simulink model "dspwavelet_frame"  (Simulink 8.3)
settings: Solver=FixedStepDiscrete  StartTime=0.0  StopTime=1024  RelTol=1e-3
model workspace: external: MAT-File dspwlets.mat (data not in the file)
undefined symbols (not defined in the file or in its folder): lod, ts
libraries: dspsigops x5, dspmlti4 x4, dspstat3 x2, simulink x2, dspmisc x1, dspsrcs4 x1
settings Model: Creator=The MathWorks Inc.  ExtModeTrigMode=oneshot  ExtModeArmWhenConnect=off
settings DataIOCC: LimitDataPoints=off  SaveOutput=off  SaveTime=off  SignalLoggingName=sigsOut
settings OptimizationCC: BlockReduction=off  BooleanDataType=off  ExpressionDepthLimit=2147483647  InitFltsAndDblsToZero=on  EfficientMapNaN2IntZero=off
settings DebuggingCC: SaveWithParameterizedLinksMsg=none  SignalResolutionControl=TryResolveAllWithWarning  SolverPrmCheckMsg=none  MultiTaskDSMMsg=warning  MultiTaskCondExecSysMsg=none  IntegerOverflowMsg=none  FcnCallInpInsideContextMsg=UseLocalSettings  StrictBusMsg=None
settings HardwareCC: TargetUnknown=on
settings RTWCC: IncludeERTFirstTime=on
settings GRTTargetCC: TargetFcnLib=ansi_tfl_tmw.mat

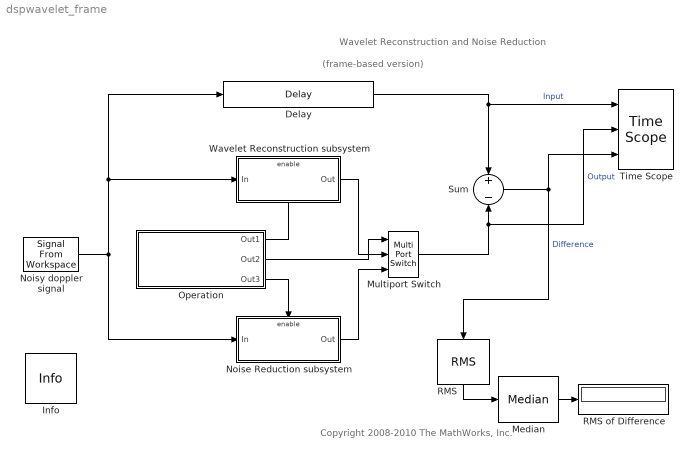
== system dspwavelet_frame ==
  note: Wavelet Reconstruction and Noise Reduction
  note: Copyright 2008-2010 The MathWorks, Inc.
  note: (frame-based version)
  Delay : dspsigops/Delay  InputProcessing=Columns as channels (frame based)  dly_unit=Samples  delay=7*(length(lod)-1)  ic_detail=on  dif_ic_for_ch=off  dif_ic_for_dly=off  ic=0  reset_popup=None
  Info : dspmisc/Info  SystemSampleTime=-1
  Median : dspstat3/Median  sortAlg=Quick sort  directionMode=Each column  dimension=1  treatSBRowAsCol=on  outputDataTypeStr=Inherit: Same as accumulator  outputLastDataTypeStr=Inherit: Same as accumulator  outputMin=[]  outputMax=[]  accumDataTypeStr=Inherit: Same as product output  accumLastDataTypeStr=Inherit: Same as product output  roundingMode=Floor  overflowMode=off
      settings: allowOverrides=off
  Multiport Switch : MultiPortSwitch  DataPortOrder=Zero-based contiguous  Inputs=2  zeroidx=on
  Noise Reduction subsystem : Subsystem  TreatAsAtomicUnit=on
  Noisy doppler signal : dspsrcs4/Signal From Workspace  X=noisdopp  Ts=ts  nsamps=64  OutputAfterFinalValue=Setting to zero  ignoreOrWarnInputAndFrameLengths=off
  Operation : Subsystem  mask(Wavelet Application){operation=Remove noise}
      mask help: Select a wavelet application
      mask init:
      | if operation == 1
      |     str = 'Perfect Reconstruction';
      | else
      |     str = 'Remove Noise';
      | end
      mask TypeOptions operation: Perfect reconstruction | Remove noise
      mask Display: disp(str)
  RMS : dspstat3/RMS  run=on  reset_popup=None  InputProcessing=Columns as channels (frame based)  directionMode=Entire input  dimension=1  treatSBRowAsCol=on
  RMS of Difference : Display
  Sum : Sum  Inputs=+-  SaturateOnIntegerOverflow=on  InputSameDT=on  OutDataTypeStr=Inherit: Same as first input
  Time Scope : TimeScope  NumInputPorts=3  DefaultConfigurationName=spbscopes.TimeScopeBlockCfg  ScopeSpecification=DataTag4
  Wavelet Reconstruction subsystem : Subsystem  TreatAsAtomicUnit=on
  wires:
  Delay/1 -> Sum/1, Time Scope/1  "Input"
  Sum/1 -> RMS/1, Time Scope/3  "Difference"
  Operation/1(Out1) -> Wavelet Reconstruction subsystem/Enable
  Noisy doppler signal/1 -> Noise Reduction subsystem/1(In), Delay/1, Wavelet Reconstruction subsystem/1(In)
  Operation/2(Out2) -> Multiport Switch/1
  Operation/3(Out3) -> Noise Reduction subsystem/Enable
  Noise Reduction subsystem/1(Out) -> Multiport Switch/3
  Multiport Switch/1 -> Time Scope/2, Sum/2  "Output"
  RMS/1 -> Median/1
  Wavelet Reconstruction subsystem/1(Out) -> Multiport Switch/2
  Median/1 -> RMS of Difference/1

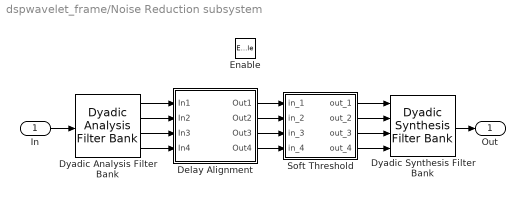
== system dspwavelet_frame/Noise Reduction subsystem ==
  In : Inport
  Enable : EnablePort
  Delay Alignment : Subsystem
  Dyadic Analysis Filter Bank : dspmlti4/Dyadic Analysis Filter Bank  Wname=User-defined  OrdRec_ordDec=[1 / 1]  Order=2  LPF=lod  HPF=hid  NumLevels=3  tree=Asymmetric  Output=Multiple ports
  Dyadic Synthesis Filter Bank : dspmlti4/Dyadic Synthesis Filter Bank  Wname=User-defined  OrdRec_ordDec=[1 / 1]  Order=2  LPF=lor  HPF=hir  NumLevels=3  tree=Asymmetric  Input=Multiple ports
  Soft Threshold : Subsystem  mask(Soft Threshold){st=[3 2 1 0]}
      mask prompts: st "Vector of thresholds for each level:"
      mask help: Apply a soft threshold (deadzone transfer function) to each signal in the decomposition. First threshold applies to top-most filter bank output.
      mask init:
      | x=([-1 1 NaN 0 0 NaN -1 -.5 .5 1]+1)/2*.7+.15;
      | y=([0 0 NaN -1 1 NaN -1 0 0 1]+1)/2*.7+.05;
      mask Help: Vector of thresholds for each decomposition level.
      mask Display:
      | text(.1,.9,'Dead Zone')
      | plot(x,y)
  Out : Outport
  wires:
  In/1 -> Dyadic Analysis Filter Bank/1
  Dyadic Synthesis Filter Bank/1 -> Out/1
  Dyadic Analysis Filter Bank/2 -> Delay Alignment/2(In2)
  Dyadic Analysis Filter Bank/1 -> Delay Alignment/1(In1)
  Delay Alignment/2(Out2) -> Soft Threshold/2(in_2)
  Delay Alignment/1(Out1) -> Soft Threshold/1(in_1)
  Soft Threshold/1(out_1) -> Dyadic Synthesis Filter Bank/1
  Soft Threshold/2(out_2) -> Dyadic Synthesis Filter Bank/2
  Dyadic Analysis Filter Bank/3 -> Delay Alignment/3(In3)
  Dyadic Analysis Filter Bank/4 -> Delay Alignment/4(In4)
  Delay Alignment/3(Out3) -> Soft Threshold/3(in_3)
  Delay Alignment/4(Out4) -> Soft Threshold/4(in_4)
  Soft Threshold/3(out_3) -> Dyadic Synthesis Filter Bank/3
  Soft Threshold/4(out_4) -> Dyadic Synthesis Filter Bank/4

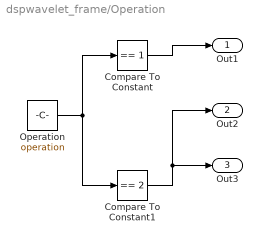
== system dspwavelet_frame/Operation ==
  Compare To Constant : simulink/Logic and Bit Operations/Compare To Constant  relop===  const=1  OutDataTypeStr=uint8  ZeroCross=off
  Compare To Constant1 : simulink/Logic and Bit Operations/Compare To Constant  relop===  const=2  OutDataTypeStr=uint8  ZeroCross=off
  Operation : Constant  Value=operation
  Out1 : Outport
  Out2 : Outport  Port=2
  Out3 : Outport  Port=3
  wires:
  Operation/1 -> Compare To Constant/1, Compare To Constant1/1
  Compare To Constant/1 -> Out1/1
  Compare To Constant1/1 -> Out3/1, Out2/1

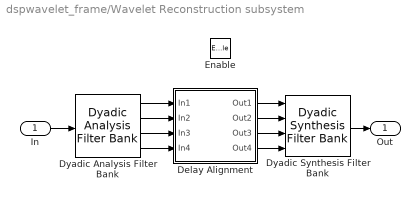
== system dspwavelet_frame/Wavelet Reconstruction subsystem ==
  In : Inport
  Enable : EnablePort
  Delay Alignment : Subsystem
  Dyadic Analysis Filter Bank : dspmlti4/Dyadic Analysis Filter Bank  Wname=User-defined  OrdRec_ordDec=[1 / 1]  Order=2  LPF=lod  HPF=hid  NumLevels=3  tree=Asymmetric  Output=Multiple ports
  Dyadic Synthesis Filter Bank : dspmlti4/Dyadic Synthesis Filter Bank  Wname=User-defined  OrdRec_ordDec=[1 / 1]  Order=2  LPF=lor  HPF=hir  NumLevels=3  tree=Asymmetric  Input=Multiple ports
  Out : Outport
  wires:
  In/1 -> Dyadic Analysis Filter Bank/1
  Dyadic Synthesis Filter Bank/1 -> Out/1
  Dyadic Analysis Filter Bank/2 -> Delay Alignment/2(In2)
  Dyadic Analysis Filter Bank/1 -> Delay Alignment/1(In1)
  Delay Alignment/2(Out2) -> Dyadic Synthesis Filter Bank/2
  Delay Alignment/1(Out1) -> Dyadic Synthesis Filter Bank/1
  Dyadic Analysis Filter Bank/3 -> Delay Alignment/3(In3)
  Dyadic Analysis Filter Bank/4 -> Delay Alignment/4(In4)
  Delay Alignment/3(Out3) -> Dyadic Synthesis Filter Bank/3
  Delay Alignment/4(Out4) -> Dyadic Synthesis Filter Bank/4

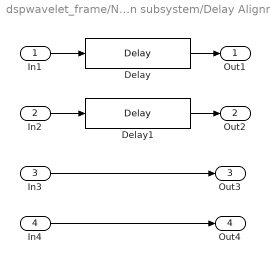
== system dspwavelet_frame/Noise Reduction subsystem/Delay Alignment ==
  In1 : Inport
  In2 : Inport  Port=2
  In3 : Inport  Port=3
  In4 : Inport  Port=4
  Delay : dspsigops/Delay  InputProcessing=Columns as channels (frame based)  dly_unit=Samples  delay=3*(length(lod)-1)  ic_detail=on  dif_ic_for_ch=off  dif_ic_for_dly=off  ic=0  reset_popup=None
  Delay1 : dspsigops/Delay  InputProcessing=Columns as channels (frame based)  dly_unit=Samples  delay=length(lod) - 1  ic_detail=on  dif_ic_for_ch=off  dif_ic_for_dly=off  ic=0  reset_popup=None
  Out1 : Outport
  Out2 : Outport  Port=2
  Out3 : Outport  Port=3
  Out4 : Outport  Port=4
  wires:
  In3/1 -> Out3/1
  In4/1 -> Out4/1
  In2/1 -> Delay1/1
  Delay1/1 -> Out2/1
  In1/1 -> Delay/1
  Delay/1 -> Out1/1

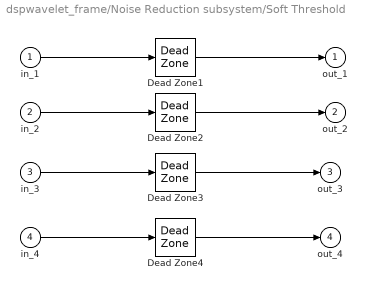
== system dspwavelet_frame/Noise Reduction subsystem/Soft Threshold ==
  in_1 : Inport
  in_2 : Inport  Port=2
  in_3 : Inport  Port=3
  in_4 : Inport  Port=4
  Dead Zone1 : DeadZone  LowerValue=-st(1)  UpperValue=st(1)  ZeroCross=off  SaturateOnIntegerOverflow=on
  Dead Zone2 : DeadZone  LowerValue=-st(2)  UpperValue=st(2)  ZeroCross=off  SaturateOnIntegerOverflow=on
  Dead Zone3 : DeadZone  LowerValue=-st(3)  UpperValue=st(3)  ZeroCross=off  SaturateOnIntegerOverflow=on
  Dead Zone4 : DeadZone  LowerValue=-st(4)  UpperValue=st(4)  ZeroCross=off  SaturateOnIntegerOverflow=on
  out_1 : Outport
  out_2 : Outport  Port=2
  out_3 : Outport  Port=3
  out_4 : Outport  Port=4
  wires:
  in_1/1 -> Dead Zone1/1
  in_2/1 -> Dead Zone2/1
  in_3/1 -> Dead Zone3/1
  in_4/1 -> Dead Zone4/1
  Dead Zone1/1 -> out_1/1
  Dead Zone2/1 -> out_2/1
  Dead Zone3/1 -> out_3/1
  Dead Zone4/1 -> out_4/1

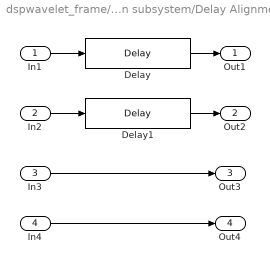
== system dspwavelet_frame/Wavelet Reconstruction subsystem/Delay Alignment ==
  In1 : Inport
  In2 : Inport  Port=2
  In3 : Inport  Port=3
  In4 : Inport  Port=4
  Delay : dspsigops/Delay  InputProcessing=Columns as channels (frame based)  dly_unit=Samples  delay=3*(length(lod)-1)  ic_detail=on  dif_ic_for_ch=off  dif_ic_for_dly=off  ic=0  reset_popup=None
  Delay1 : dspsigops/Delay  InputProcessing=Columns as channels (frame based)  dly_unit=Samples  delay=length(lod) - 1  ic_detail=on  dif_ic_for_ch=off  dif_ic_for_dly=off  ic=0  reset_popup=None
  Out1 : Outport
  Out2 : Outport  Port=2
  Out3 : Outport  Port=3
  Out4 : Outport  Port=4
  wires:
  In3/1 -> Out3/1
  In4/1 -> Out4/1
  In2/1 -> Delay1/1
  Delay1/1 -> Out2/1
  In1/1 -> Delay/1
  Delay/1 -> Out1/1
